simulink model "PMSM_FOC_Speed_PR"  (R2024b)
settings: Solver=FixedStepAuto  StartTime=0.0  StopTime=1  FixedStep=1e-6  RelTol=1e-3
model workspace (MAT data in the model file):
  B = 0
  Current_Filter_On = 0
  F = 10000
  J = 5.8e-05
  Ls = 0.0005125
  PR_ki = 150
  PR_wc = 150
  Pn = 5
  Rs = 0.1445
  T_deadband = 3e-06
  Ts = 5e-05
  Vdc = 60
  id_ki = 0.8
  id_kp = 0.6
  iq_ki = 0.8
  iq_kp = 0.7
  psi_f = 0.0113
  speed_ki = 1.2
  speed_kp = 0.7
undefined symbols (not defined in the file): sigbuilder_block
libraries: simulink x2, spsDCVoltageSourceLib x1, spsOnDelayLib x1, spsPermanentMagnetSynchronousMachineLib x1, slpidlib x1, spsTwoLevelConverterLib x1, spspowerguiLib x1
settings Model: Creator=A  LastModifiedBy=31904
settings OptimizationCC: ReuseModelBlockBuffer=off
settings ModelReferenceCC: EnableRefExpFcnMdlSchedulingChecks=on
settings RTWCC: GPUComputeCapability=3.5

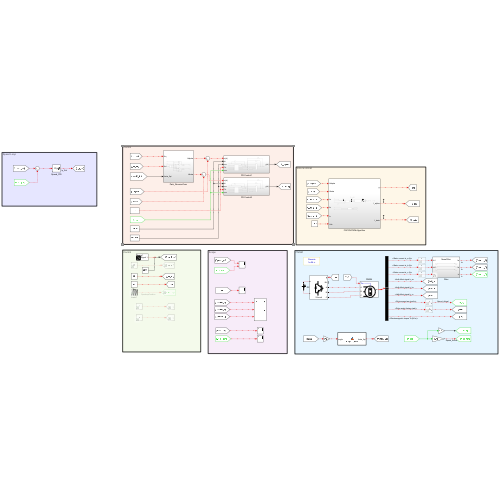
[thumbnail: Simulink's stored preview of the top-level diagram]
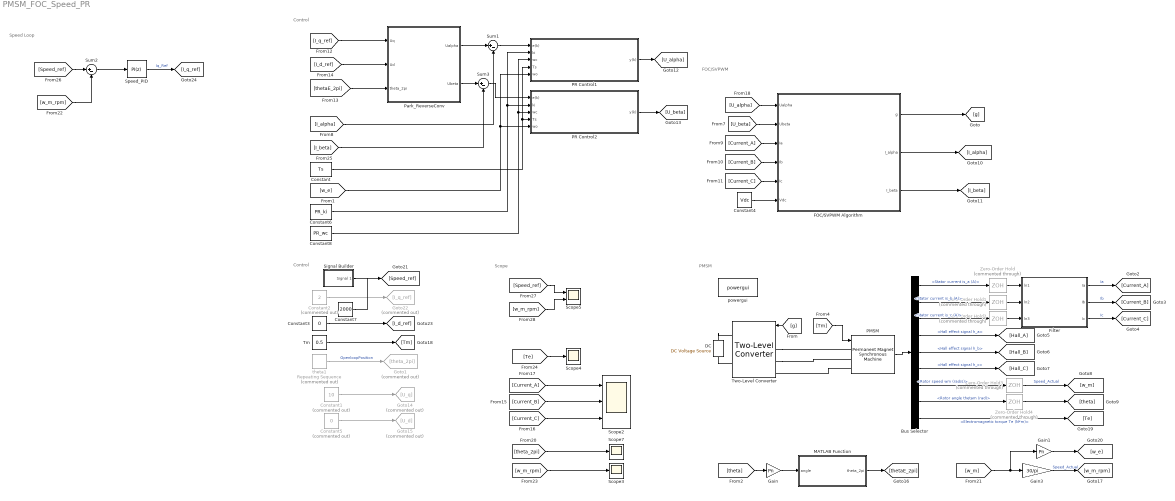
== system PMSM_FOC_Speed_PR ==
  note: Speed Loop
  note: Control
  note: Scope
  note: Control
  note: FOC/SVPWM
  note: PMSM
  Bus Selector : BusSelector  OutputSignals=Stator current is_a (A),Stator current is_b (A),Stator current is_c (A),Hall effect signal h_a,Hall effect signal h_b,Hall effect signal h_c,Rotor speed wm (rad/s),Rotor angle thetam (rad),Electromagnetic torque Te (N*m)
  Constant : Constant  Value=Ts
  Constant1 : Constant  Commented=on  Value=10
  Constant2 : Constant  Commented=on  Value=2
  Constant3 : Constant  Value=0
  Constant4 : Constant  Value=Vdc
  Constant5 : Constant  Commented=on  Value=0
  Constant6 : Constant  Value=PR_ki
  Constant7 : Constant  Value=2000
  Constant8 : Constant  Value=PR_wc
  DC : spsDCVoltageSourceLib/DC Voltage Source  Amplitude=Vdc  Measurements=None
  FOC/SVPWM Algorithm : Subsystem
  Filter : Subsystem  Variant=on
  Gain : Gain  Gain=Pn
  Gain1 : Gain  Gain=Pn
  Gain3 : Gain  Gain=30/pi
  Goto1 : Goto  Commented=on  GotoTag=theta_2pi
  Goto14 : Goto  Commented=on  GotoTag=U_q
  Goto15 : Goto  Commented=on  GotoTag=U_d
  Goto22 : Goto  Commented=on  GotoTag=I_q_ref
  MATLAB Function : MATLAB Function  TreatAsAtomicUnit=on
  PMSM : spsPermanentMagnetSynchronousMachineLib/Permanent Magnet Synchronous Machine  NbPhases=3  FluxDistribution=Sinusoidal  RotorType=Round  MechanicalLoad=Torque Tm  PresetModel=No  ShowDetailedParameters=on  MeasurementBus=off  Resistance=Rs  Inductance=8.5e-3  dqInductances=[8.5e-3,8.5e-3]  La=Ls  MachineConstant=Flux linkage established by magnets (V.s)  Flux=psi_f  VoltageCst=10.248  TorqueCst=0.08475  Flat=120  Mechanical=[J B Pn 0]  PolePairs=4  InitialConditions=[0,0, 0,0]  InitialConditions5ph=[0 0 0 0 0 0]  RefAngle=Aligned with phase A axis (original Park)  IterativeDiscreteModel=Trapezoidal non iterative  TsBlock=-1  TsPowergui=0
  PR Control1 : Subsystem
  PR Control2 : Subsystem
  Park_ReverseConv : Subsystem
  Scope2 : Scope  NumInputPorts=3
  Scope3 : Scope
  Scope4 : Scope
  Scope5 : Scope  NumInputPorts=2
  Scope7 : Scope
  Signal Builder : Subsystem  Tag=STV Subsys  LoadFcn=sigbuilder_block('load');  StartFcn=sigbuilder_block('start');  StopFcn=sigbuilder_block('stop');  ClipboardFcn=sigbuilder_block('clipboard');  mask(Sigbuilder block){tuvar=[0:10]}
      mask help: Simulink:masks:SigbuilderBlock_MD
      mask init:
      | if ~strcmp(get_param(bdroot(gcbh),'SimulationStatus'),'stopped') tuvar = sigbuilder_block('maskInit'); end
      settings: CopyFcn=sigbuilder_block('copy');  DeleteFcn=sigbuilder_block('delete');  ModelCloseFcn=sigbuilder_block('modelClose');  PreSaveFcn=sigbuilder_block('preSave');  PauseFcn=sigbuilder_block('pause');  ContinueFcn=sigbuilder_block('continue');  NameChangeFcn=sigbuilder_block('namechange');  OpenFcn=sigbuilder_block('open',[458.1 40.8 550.2 399.9 ]);  CloseFcn=sigbuilder_block('close');
      mask Display: plot(0, 0, 100, 100,[2, 2, 32, 32, 2], [68, 8, 8, 68, 68],[32, 2], [38, 38], [32, 19, 2],[53, 60, 44], [32, 17, 17, 2],[16, 16, 31, 31]);txt = getActiveGroup(gcbh);text(2, 100, txt,'verticalAlignment', 'top');
  Speed_PID : slpidlib/PID Controller  Controller=PI  Form=Parallel  TimeDomain=Discrete-time  UseExternalTs=off  SampleTime=-1  IntegratorMethod=Forward Euler  FilterMethod=Forward Euler  ControllerParametersSource=internal  P=speed_kp  I=speed_ki  UseKiTs=off  D=0  UseExternalDerivativeSource=off  N=100  UseFilter=on  TunerSelectOption=Transfer Function Based (PID Tuner App)  InitialConditionSource=internal  InitialConditionForIntegrator=0  InitialConditionForFilter=0  DifferentiatorICPrevScaledInput=0  ExternalReset=none  TrackingMode=off  Kt=1  LimitOutput=on  SatLimitsSource=internal  UpperSaturationLimit=Vdc  LowerSaturationLimit=-Vdc  LinearizeAsGain=on  AntiWindupMode=back-calculation  Kb=0.5  LimitIntegrator=off  UpperIntegratorSaturationLimit=inf  LowerIntegratorSaturationLimit=-inf  POutMin=[]  POutMax=[]  IOutMin=[]  IOutMax=[]  DOutMin=[]  DOutMax=[]  NOutMin=[]  NOutMax=[]  SumOutMin=[]  SumOutMax=[]  SaturationOutMin=[]  SaturationOutMax=[]  PParamMin=[]  PParamMax=[]  IParamMin=[]  IParamMax=[]  DParamMin=[]  DParamMax=[]  NParamMin=[]  NParamMax=[]  KbParamMin=[]  KbParamMax=[]  KtParamMin=[]  KtParamMax=[]  KbOutMin=[]  KbOutMax=[]  KtOutMin=[]  KtOutMax=[]  IntegratorOutMin=[]  IntegratorOutMax=[]  FilterOutMin=[]  FilterOutMax=[]  SumI1OutMin=[]  SumI1OutMax=[]  SumI2OutMin=[]  SumI2OutMax=[]  SumI3OutMin=[]  SumI3OutMax=[]  SumI4OutMin=[]  SumI4OutMax=[]  SumDOutMin=[]  SumDOutMax=[]  DifferentiatorOutMin=[]  DifferentiatorOutMax=[]  FilterDiffOutCoefMin=[]  FilterDiffOutCoefMax=[]  ReciprocalOutMin=[]  ReciprocalOutMax=[]  SumDenOutMin=[]  SumDenOutMax=[]  SumNumOutMin=[]  SumNumOutMax=[]  DivideOutMin=[]  DivideOutMax=[]  UdiffTsProdOutMin=[]  UdiffTsProdOutMax=[]  NTsProdOutMin=[]  NTsProdOutMax=[]  UintegralTsProdOutMin=[]  UintegralTsProdOutMax=[]  UngainTsProdOutMin=[]  UngainTsProdOutMax=[]  ClampingZeroOutDataTypeStr=Inherit: Inherit via back propagation  ClampingZeroOutMin=[]  ClampingZeroOutMax=[]  FilterDenConstantOutDataTypeStr=Inherit: Inherit via back propagation  FilterDenConstantOutMin=[]  FilterDenConstantOutMax=[]  PCopyOutDataTypeStr=Inherit: Inherit via back propagation  PCopyOutMin=[]  PCopyOutMax=[]  NCopyOutDataTypeStr=Inherit: Inherit via back propagation  NCopyOutMin=[]  NCopyOutMax=[]  IntegratorContinuousStateAttributes=''  IntegratorStateMustResolveToSignalObject=off  IntegratorRTWStateStorageClass=Auto  FilterContinuousStateAttributes=''  FilterStateMustResolveToSignalObject=off  FilterRTWStateStorageClass=Auto  ParallelPVariant=InternalParameters  IdealPVariant=Disabled  IVariant=InternalParameters  DVariant=Disabled  IntegratorVariant=Discrete  SatVariant=Enabled  AWVariant=BackCalculation  PCopyVariant=Disabled  TRVariant=Disabled  FdbkBlocksVariant=Forward  IdealPFdbkVariant=Disabled  SatFdbkVariant=Disabled  DerivativeFilterVariant=Disabled  NVariant=Disabled  NCopyVariant=Disabled_SignalSpec  FilterICVariant=Disabled  IntegratorICVariant=InternalICs  ExternalResetVariant=Disabled  TRSumVariant=Passthrough  SumFdbkVariant=Disabled  SumVariant=Sum_PI  TsampFilterVariant=InternalTs  TsampNgainVariant=Passthrough  TsampIntegralVariant=Disabled_SignalSpec  ExternalSaturationOutDataTypeStr=Inherit: Same as second input  DerivativeSourceVariant=Disabled  PreIntVariant=InternalPreInt
  Sum1 : Sum  Inputs=|+-
  Sum2 : Sum  Inputs=|+-
  Sum3 : Sum  Inputs=|+-
  Tm : Constant  Value=0.5
  Two-Level Converter : spsTwoLevelConverterLib/Two-Level Converter  ModelType=Switching devices  Ron=1e-3  Rs=1e6  Cs=inf  Vforward=[0,0]  Ron_Diode=1e-3  Rs_Diode=1e6  Cs_Diode=inf  Vf_Diode=1e-3  Rs_CurrentSource=inf  Ron_ACsource=1e-3
  Zero-Order Hold{,1..4} (5 alike) : ZeroOrderHold  Commented=through  SampleTime=1/F
  powergui : spspowerguiLib/powergui  Priority=1  SimulationMode=Discrete  SampleTime=1e-6  frequency=60  Iterations=50  frequencyindice=0  Pbase=100e6  ErrMax=1e-4  UnitsV=kV  UnitsW=MW  buscounter=0  FunctionMessages=off  echomessages=off  EnableUseOfTLC=off  CurrentSourceSwitches=off  DisableSnubberDevices=off  DisableRonSwitches=off  DisableVfSwitches=off  DisplayEquations=off  AutomaticDiscreteSolvers=off  SolverType=Tustin/Backward Euler (TBE)  Interpol=off  ExternalGateDelay=off  methode=off  Ts=100  x0status=blocks  SPID=on  SwTol=0  HookPort=off  NonlinearTolerance=1e-4  nMaxIteration=100  ContinueOnMaxIteration=off  RestoreLinks=warning  ResistiveCurrentMeasurement=off  Frange=[0:2:500]  Ylog=off  Xlog=on  ShowGrid=off  save=off  variable=ZData  structure=0  ZoomFFT=off  StartTime=0.0  cycles=1  DisplayStyle=1  fundamental=60  FreqAxis=off  MaxFrequency=1000  frequencyindicesteady=1  RmsSteady=1  display=off
  theta1 : simulink/Sources/Repeating Sequence  Commented=on  rep_seq_t=[0 0.1]  rep_seq_y=[0 2*pi]
  wires:
  Constant4/1 -> FOC/SVPWM Algorithm/6(Vdc)
  FOC/SVPWM Algorithm/3(I_beta) -> [I_beta]
  [U_beta] -> FOC/SVPWM Algorithm/2(Ubeta)
  [U_alpha] -> FOC/SVPWM Algorithm/1(Ualpha)
  [Current_A] -> FOC/SVPWM Algorithm/3(Ia)
  [Current_C] -> FOC/SVPWM Algorithm/5(Ic)
  FOC/SVPWM Algorithm/2(I_alpha) -> [I_alpha]
  [Current_B] -> FOC/SVPWM Algorithm/4(Ib)
  Zero-Order Hold4/1 -> [theta]
  Bus Selector/1 -> Zero-Order Hold/1  "<Stator current is_a (A)>"
  Zero-Order Hold/1 -> Filter/1(ln1)
  Zero-Order Hold1/1 -> Filter/2(ln2)
  Bus Selector/4 -> [Hall_A]  "<Hall effect signal h_a>"
  [theta] -> Gain/1
  Bus Selector/2 -> Zero-Order Hold1/1  "<Stator current is_b (A)>"
  [g] -> Two-Level Converter/1
  Bus Selector/3 -> Zero-Order Hold2/1  "<Stator current is_c (A)>"
  [Tm] -> PMSM/1
  Zero-Order Hold3/1 -> [w_m]  "Speed_Actual"
  Bus Selector/8 -> Zero-Order Hold4/1  "<Rotor angle thetam (rad)>"
  MATLAB Function/1(theta_2pi) -> [thetaE_2pi]
  Bus Selector/7 -> Zero-Order Hold3/1  "<Rotor speed wm (rad/s)>"
  PMSM/1 -> Bus Selector/1
  Bus Selector/5 -> [Hall_B]  "<Hall effect signal h_b>"
  Zero-Order Hold2/1 -> Filter/3(ln3)
  Bus Selector/6 -> [Hall_C]  "<Hall effect signal h_c>"
  Constant3/1 -> [I_d_ref]
  Constant2/1 -> Goto22/1
  [I_q_ref] -> Park_ReverseConv/1(Uq)
  [Current_C] -> Scope2/3
  [Current_B] -> Scope2/2
  [Current_A] -> Scope2/1
  [theta_2pi] -> Scope7/1
  Filter/1(Ia) -> [Current_A]  "Ia"
  Filter/2(Ib) -> [Current_B]  "Ib"
  Filter/3(Ic) -> [Current_C]  "Ic"
  FOC/SVPWM Algorithm/1(g) -> [g]
  theta1/1 -> Goto1/1  "OpenloopPosition"
  [I_d_ref] -> Park_ReverseConv/2(Ud)
  Constant5/1 -> Goto15/1
  Constant1/1 -> Goto14/1
  [w_m] -> Gain1/1, Gain3/1
  Gain3/1 -> [w_m_rpm]  "Speed_Actual"
  [w_m_rpm] -> Scope3/1
  Gain/1 -> MATLAB Function/1(angle)
  Tm/1 -> [Tm]
  Bus Selector/9 -> [Te]  "<Electromagnetic torque Te (N*m)>"
  [Te] -> Scope4/1
  PR Control2/1(y(k)) -> [U_beta]
  PR Control1/1(y(k)) -> [U_alpha]
  Constant7/1 -> [Speed_ref]
  Sum2/1 -> Speed_PID/1
  [w_m_rpm] -> Sum2/2
  [Speed_ref] -> Sum2/1
  Speed_PID/1 -> [I_q_ref]  "Iq_Ref"
  [Speed_ref] -> Scope5/1
  [w_m_rpm] -> Scope5/2
  Signal Builder/1(Signal 1) -> ?
  [thetaE_2pi] -> Park_ReverseConv/3(theta_2pi)
  Park_ReverseConv/1(Ualpha) -> Sum1/1
  Park_ReverseConv/2(Ubeta) -> Sum3/1
  Sum1/1 -> PR Control1/1(e(k))
  [I_alpha] -> Sum1/2
  [I_beta] -> Sum3/2
  Sum3/1 -> PR Control2/1(e(k))
  Constant/1 -> PR Control1/4(Ts), PR Control2/4(Ts)
  Constant6/1 -> PR Control1/2(ki), PR Control2/2(ki)
  Constant8/1 -> PR Control1/3(wc), PR Control2/3(wc)
  Gain1/1 -> [w_e]
  [w_e] -> PR Control1/5(wo), PR Control2/5(wo)
  connections:
  DC/LConn1 -- Two-Level Converter/RConn2
  DC/RConn1 -- Two-Level Converter/RConn1
  PMSM/LConn3 -- Two-Level Converter/LConn3
  Two-Level Converter/LConn1 -- PMSM/LConn1
  Two-Level Converter/LConn2 -- PMSM/LConn2

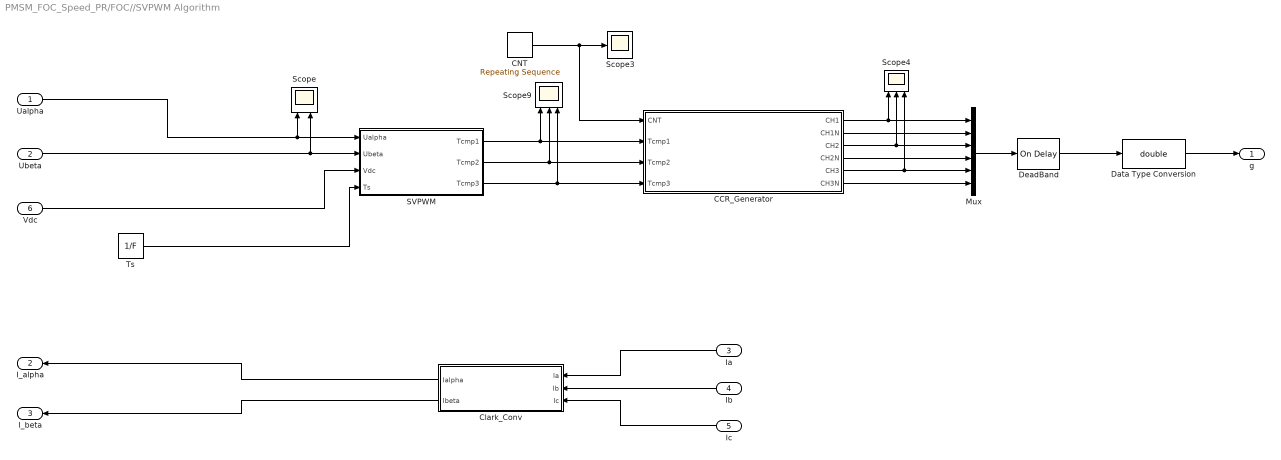
== system PMSM_FOC_Speed_PR/FOC//SVPWM Algorithm ==
  Ualpha : Inport
  Ubeta : Inport  Port=2
  Ia : Inport  Port=3
  Ib : Inport  Port=4
  Ic : Inport  Port=5
  Vdc : Inport  Port=6
  CCR_Generator : MATLAB Function  TreatAsAtomicUnit=on
  CNT : simulink/Sources/Repeating Sequence  rep_seq_t=[0 1/(2*F) 1/F]  rep_seq_y=[0 1/(2*F) 0]
  Clark_Conv : Subsystem
  Data Type Conversion : DataTypeConversion  OutDataTypeStr=double  SaturateOnIntegerOverflow=off  RndMeth=Floor
  DeadBand : spsOnDelayLib/On Delay  DelayType=On delay  delay=T_deadband  ic=0  Ts=0
  Mux : Mux  Inputs=6
  SVPWM : Subsystem
  Scope : Scope  NumInputPorts=2
  Scope3 : Scope
  Scope4 : Scope  NumInputPorts=3
  Scope9 : Scope  NumInputPorts=3
  Ts : Constant  Value=1/F
  g : Outport
  I_alpha : Outport  Port=2
  I_beta : Outport  Port=3
  wires:
  SVPWM/3(Tcmp3) -> CCR_Generator/4(Tcmp3), Scope9/3
  Clark_Conv/1(Ialpha) -> I_alpha/1
  CCR_Generator/3(CH2) -> Mux/3, Scope4/2
  SVPWM/2(Tcmp2) -> CCR_Generator/3(Tcmp2), Scope9/2
  CCR_Generator/2(CH1N) -> Mux/2
  CCR_Generator/5(CH3) -> Mux/5, Scope4/3
  SVPWM/1(Tcmp1) -> CCR_Generator/2(Tcmp1), Scope9/1
  Clark_Conv/2(Ibeta) -> I_beta/1
  CCR_Generator/4(CH2N) -> Mux/4
  Ualpha/1 -> SVPWM/1(Ualpha), Scope/1
  CCR_Generator/6(CH3N) -> Mux/6
  Mux/1 -> DeadBand/1
  Ubeta/1 -> Scope/2, SVPWM/2(Ubeta)
  CNT/1 -> Scope3/1, CCR_Generator/1(CNT)
  CCR_Generator/1(CH1) -> Mux/1, Scope4/1
  Data Type Conversion/1 -> g/1
  Vdc/1 -> SVPWM/3(Vdc)
  Ic/1 -> Clark_Conv/3(Ic)
  Ib/1 -> Clark_Conv/2(Ib)
  Ia/1 -> Clark_Conv/1(Ia)
  Ts/1 -> SVPWM/4(Ts)
  DeadBand/1 -> Data Type Conversion/1

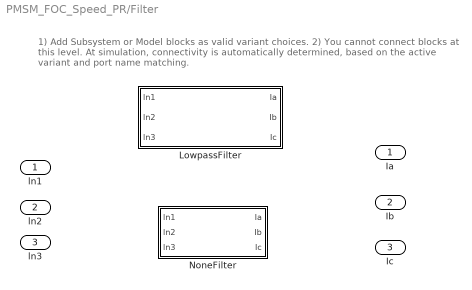
== system PMSM_FOC_Speed_PR/Filter ==
  note: 1) Add Subsystem or Model blocks as valid variant choices.
      | 2) You cannot connect blocks at this level. At simulation, connectivity is automatically
      | determined, based on the active variant and port name matching.
  ln1 : Inport
  ln2 : Inport  Port=2
  ln3 : Inport  Port=3
  LowpassFilter : Subsystem  VariantControl=Current_Filter_On==1
  NoneFilter : Subsystem  VariantControl=Current_Filter_On==0
  Ia : Outport
  Ib : Outport  Port=2
  Ic : Outport  Port=3

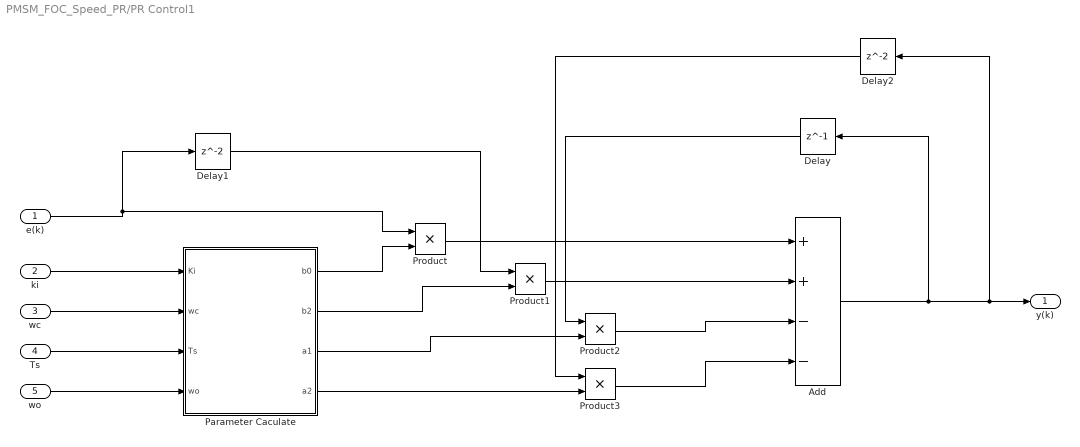
== system PMSM_FOC_Speed_PR/PR Control1 ==
  e(k) : Inport
  ki : Inport  Port=2
  wc : Inport  Port=3
  Ts : Inport  Port=4
  wo : Inport  Port=5
  Add : Sum  Inputs=++--
  Delay : Delay  DelayLength=1  InputProcessing=Columns as channels (frame based)
  Delay1 : Delay  InputProcessing=Columns as channels (frame based)
  Delay2 : Delay  InputProcessing=Columns as channels (frame based)
  Parameter Caculate : MATLAB Function  TreatAsAtomicUnit=on
  Product{,1..3} (4 alike) : Product
  y(k) : Outport
  wires:
  Ts/1 -> Parameter Caculate/3(Ts)
  wc/1 -> Parameter Caculate/2(wc)
  wo/1 -> Parameter Caculate/4(wo)
  Product2/1 -> Add/3
  ki/1 -> Parameter Caculate/1(Ki)
  Parameter Caculate/4(a2) -> Product3/2
  Delay2/1 -> Product3/1
  Parameter Caculate/1(b0) -> Product/2
  Delay/1 -> Product2/1
  Parameter Caculate/2(b2) -> Product1/2
  Add/1 -> Delay2/1, y(k)/1, Delay/1
  Product3/1 -> Add/4
  Product/1 -> Add/1
  Product1/1 -> Add/2
  e(k)/1 -> Product/1, Delay1/1
  Delay1/1 -> Product1/1
  Parameter Caculate/3(a1) -> Product2/2

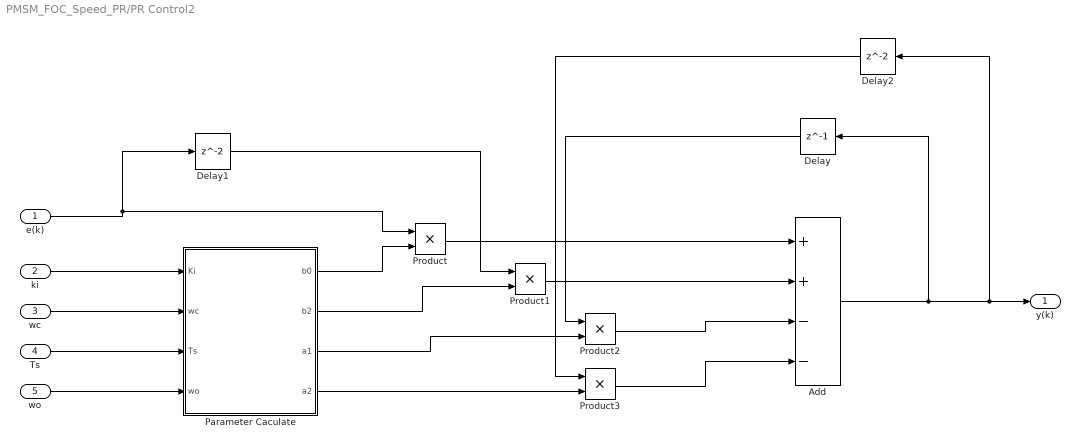
== system PMSM_FOC_Speed_PR/PR Control2 ==
  e(k) : Inport
  ki : Inport  Port=2
  wc : Inport  Port=3
  Ts : Inport  Port=4
  wo : Inport  Port=5
  Add : Sum  Inputs=++--
  Delay : Delay  DelayLength=1  InputProcessing=Columns as channels (frame based)
  Delay1 : Delay  InputProcessing=Columns as channels (frame based)
  Delay2 : Delay  InputProcessing=Columns as channels (frame based)
  Parameter Caculate : MATLAB Function  TreatAsAtomicUnit=on
  Product{,1..3} (4 alike) : Product
  y(k) : Outport
  wires:
  Parameter Caculate/3(a1) -> Product2/2
  Delay1/1 -> Product1/1
  e(k)/1 -> Delay1/1, Product/1
  Product1/1 -> Add/2
  Product/1 -> Add/1
  Product3/1 -> Add/4
  Add/1 -> Delay/1, y(k)/1, Delay2/1
  Parameter Caculate/2(b2) -> Product1/2
  Delay/1 -> Product2/1
  Parameter Caculate/1(b0) -> Product/2
  Delay2/1 -> Product3/1
  Parameter Caculate/4(a2) -> Product3/2
  ki/1 -> Parameter Caculate/1(Ki)
  Product2/1 -> Add/3
  wo/1 -> Parameter Caculate/4(wo)
  wc/1 -> Parameter Caculate/2(wc)
  Ts/1 -> Parameter Caculate/3(Ts)

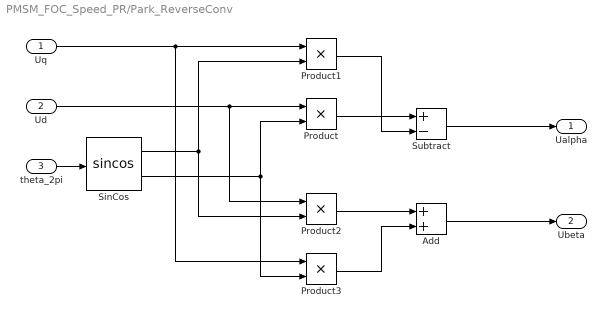
== system PMSM_FOC_Speed_PR/Park_ReverseConv ==
  Uq : Inport
  Ud : Inport  Port=2
  theta_2pi : Inport  Port=3
  Add : Sum
  Product{,1..3} (4 alike) : Product
  SinCos : Trigonometry  Operator=sincos
  Subtract : Sum  Inputs=+-
  Ualpha : Outport
  Ubeta : Outport  Port=2
  wires:
  Uq/1 -> Product3/1, Product1/1
  Ud/1 -> Product2/1, Product/1
  SinCos/2 -> Product3/2, Product/2
  Product/1 -> Subtract/1
  SinCos/1 -> Product2/2, Product1/2
  Product1/1 -> Subtract/2
  Subtract/1 -> Ualpha/1
  Product2/1 -> Add/1
  Product3/1 -> Add/2
  Add/1 -> Ubeta/1
  theta_2pi/1 -> SinCos/1

== system PMSM_FOC_Speed_PR/Signal Builder ==
  Demux : Demux  Tag=STV Demux  Outputs=1
      settings: DisplayOption=none
  FromWs : FromWorkspace  Tag=STV FromWs  VariableName=tuvar
      SigBuilderData=|
      | common.afterFinalStr = 'Extrapolate'
      | common.sampleTime = 0
      | dataSet.timeRange = [0 1]
      | dataSet.name = 'Group 1'
      | sbobj.Groups.Name = 'Group 1'
      | sbobj.Groups.Signals.Name = 'Signal 1'
      | sbobj.Groups.Signals.XData = [0 0 0.2 0.2 0.3 0.3 0.5 0.5 0.6 0.6 0.8 0.8 0.9 0.9 1]
      | sbobj.Groups.Signals.YData = [0 1000 1000 3000 3000 5000 5000 4000 4000 2000 2000 1000 1000 0 0]
      | sbobj.Groups.TimeRange = [0 1]
  Signal 1 : Outport  Tag=STV Outport
  wires:
  Demux/1 -> Signal 1/1
  FromWs/1 -> Demux/1

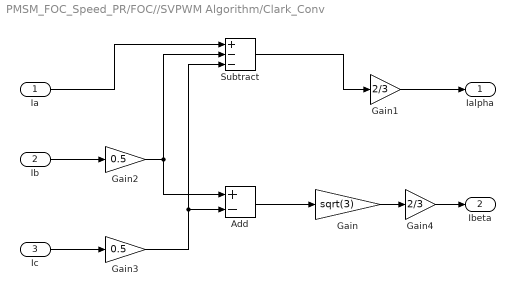
== system PMSM_FOC_Speed_PR/FOC//SVPWM Algorithm/Clark_Conv ==
  Ia : Inport
  Ib : Inport  Port=2
  Ic : Inport  Port=3
  Add : Sum  Inputs=+-  OutDataTypeStr=double
  Gain : Gain  Gain=sqrt(3)  ParamDataTypeStr=double
  Gain1 : Gain  Gain=2/3
  Gain2 : Gain  Gain=0.5
  Gain3 : Gain  Gain=0.5
  Gain4 : Gain  Gain=2/3
  Subtract : Sum  Inputs=+--  OutDataTypeStr=double
  Ialpha : Outport
  Ibeta : Outport  Port=2
  wires:
  Ia/1 -> Subtract/1
  Ib/1 -> Gain2/1
  Add/1 -> Gain/1
  Gain/1 -> Gain4/1
  Ic/1 -> Gain3/1
  Gain2/1 -> Subtract/2, Add/1
  Gain3/1 -> Subtract/3, Add/2
  Subtract/1 -> Gain1/1
  Gain1/1 -> Ialpha/1
  Gain4/1 -> Ibeta/1

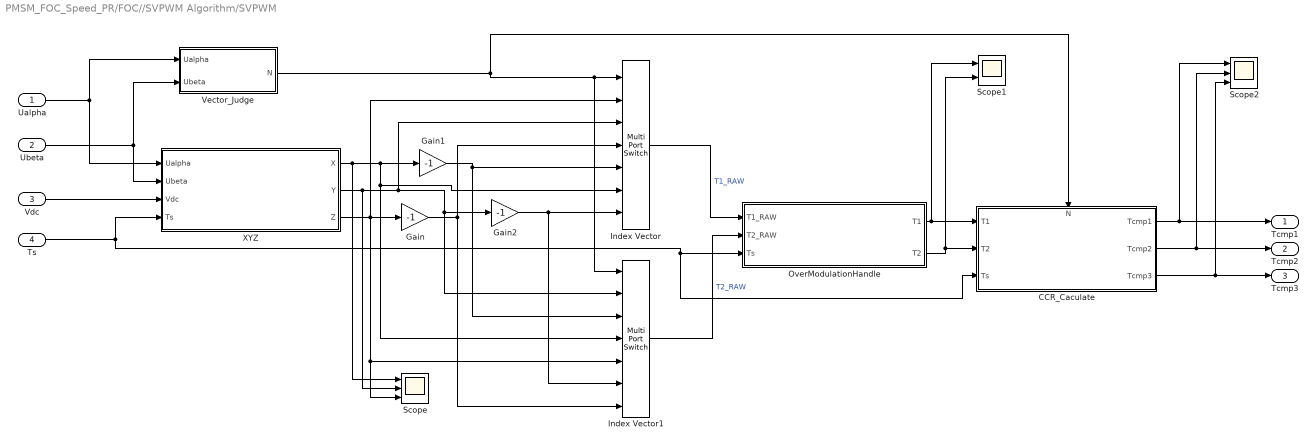
== system PMSM_FOC_Speed_PR/FOC//SVPWM Algorithm/SVPWM ==
  Ualpha : Inport
  Ubeta : Inport  Port=2
  Vdc : Inport  Port=3
  Ts : Inport  Port=4
  CCR_Caculate : Subsystem
      settings: PortSchema="{\"entries\":[{\"content\":{\"sides\":[{\"content\":{\"connectorIds\":[\"In1\",\"In2\",\"In3\"]},\"type\":\"ConnectorPlacement.EquallySpacedRectSide\",\"uuid\":\"41d89106-695f-4d7e-9c99-c52170b99868\"},{\"content\":{\"connectorIds\":[\"Out1\",\"Out2\",\"Out3\"],\"side\":\"RIGHT\"},\"type\":\"ConnectorPlacement.EquallySpacedRectSide\",\"uuid\":\"0fa1e6b9-7088-4c16-9dd3-c016449aae3e\"},{\"content\":{\"connectorIds\":[\"In4\"],\"side\":\"TOP\"},\"type\":\"ConnectorPlacement.EquallySpacedRectSide\",\"uuid\":\"6b702c00-29ab-49c7-a344-eb6fce3368af\"}]},\"type\":\"ConnectorPlacement.EquallySpacedConnector\",\"uuid\":\"c2f99839-550c-47c5-98fa-a115626cfb71\"}],\"packageUris\":[\"http://schema.mathworks.com/mf0/Connector/R2020b\"],\"version\":\"1.0\"}"
  Gain : Gain  Gain=-1
  Gain1 : Gain  Gain=-1
  Gain2 : Gain  Gain=-1
  Index Vector : MultiPortSwitch  Inputs=6  DiagnosticForDefault=None  SaturateOnIntegerOverflow=off  InputSameDT=off
  Index Vector1 : MultiPortSwitch  Inputs=6  DiagnosticForDefault=None  SaturateOnIntegerOverflow=off  InputSameDT=off
  OverModulationHandle : MATLAB Function  TreatAsAtomicUnit=on
  Scope : Scope  NumInputPorts=3
  Scope1 : Scope  NumInputPorts=2
  Scope2 : Scope  NumInputPorts=3
  Vector_Judge : Subsystem
  XYZ : Subsystem
  Tcmp1 : Outport
  Tcmp2 : Outport  Port=2
  Tcmp3 : Outport  Port=3
  wires:
  Ualpha/1 -> Vector_Judge/1(Ualpha), XYZ/1(Ualpha)
  Ubeta/1 -> Vector_Judge/2(Ubeta), XYZ/2(Ubeta)
  Vdc/1 -> XYZ/3(Vdc)
  Ts/1 -> CCR_Caculate/3(Ts), OverModulationHandle/3(Ts), XYZ/4(Ts)
  Vector_Judge/1(N) -> Index Vector1/1, Index Vector/1, CCR_Caculate/4(N)
  Index Vector1/1 -> OverModulationHandle/2(T2_RAW)  "T2_RAW"
  XYZ/3(Z) -> Scope/3, Index Vector1/5, Index Vector/2, Gain/1
  XYZ/2(Y) -> Scope/2, Index Vector1/2, Gain2/1, Index Vector/3
  Gain/1 -> Index Vector1/7, Index Vector/4
  XYZ/1(X) -> Scope/1, Index Vector1/4, Index Vector/6, Gain1/1
  Gain1/1 -> Index Vector1/3, Index Vector/5
  Gain2/1 -> Index Vector1/6, Index Vector/7
  Index Vector/1 -> OverModulationHandle/1(T1_RAW)  "T1_RAW"
  OverModulationHandle/1(T1) -> CCR_Caculate/1(T1), Scope1/1
  OverModulationHandle/2(T2) -> Scope1/2, CCR_Caculate/2(T2)
  CCR_Caculate/1(Tcmp1) -> Tcmp1/1, Scope2/1
  CCR_Caculate/2(Tcmp2) -> Tcmp2/1, Scope2/2
  CCR_Caculate/3(Tcmp3) -> Tcmp3/1, Scope2/3

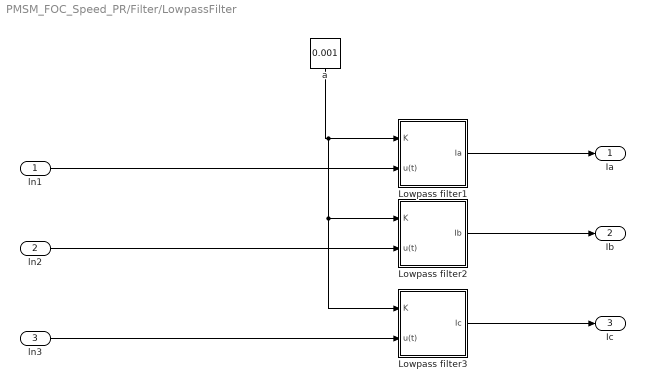
== system PMSM_FOC_Speed_PR/Filter/LowpassFilter ==
  ln1 : Inport
  ln2 : Inport  Port=2
  ln3 : Inport  Port=3
  Lowpass filter1 : Subsystem
  Lowpass filter2 : Subsystem
  Lowpass filter3 : Subsystem
  a : Constant  Value=0.001
  Ia : Outport
  Ib : Outport  Port=2
  Ic : Outport  Port=3
  wires:
  ln2/1 -> Lowpass filter2/2(u(t))
  a/1 -> Lowpass filter3/1(K), Lowpass filter2/1(K), Lowpass filter1/1(K)
  ln1/1 -> Lowpass filter1/2(u(t))
  Lowpass filter1/1(Ia) -> Ia/1
  Lowpass filter2/1(Ib) -> Ib/1
  Lowpass filter3/1(Ic) -> Ic/1
  ln3/1 -> Lowpass filter3/2(u(t))

== system PMSM_FOC_Speed_PR/Filter/NoneFilter ==
  ln1 : Inport
  ln2 : Inport  Port=2
  ln3 : Inport  Port=3
  Ia : Outport
  Ib : Outport  Port=2
  Ic : Outport  Port=3
  wires:
  ln1/1 -> Ia/1
  ln2/1 -> Ib/1
  ln3/1 -> Ic/1

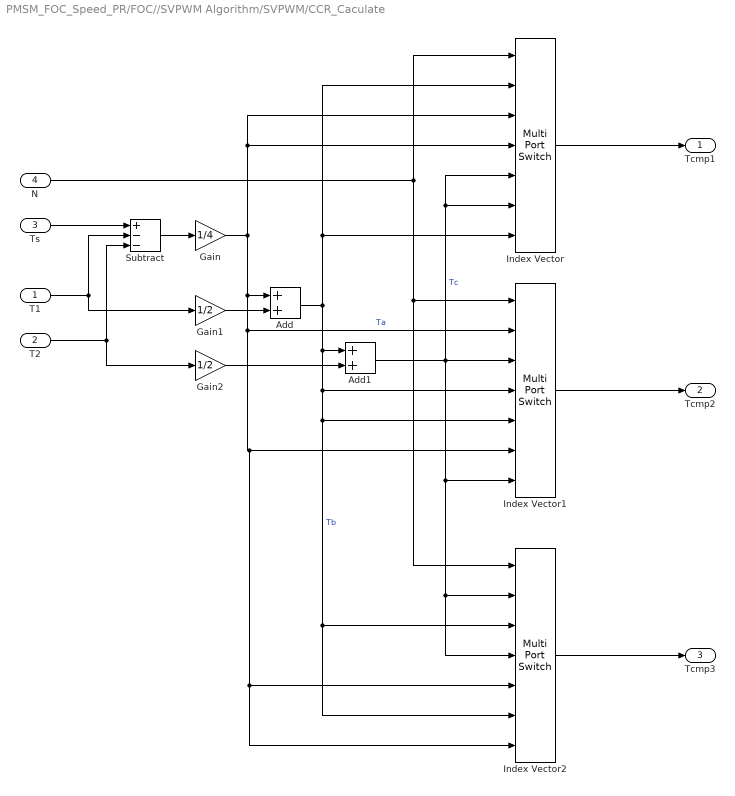
== system PMSM_FOC_Speed_PR/FOC//SVPWM Algorithm/SVPWM/CCR_Caculate ==
  T1 : Inport
  T2 : Inport  Port=2
  Ts : Inport  Port=3
  N : Inport  Port=4
  Add : Sum
  Add1 : Sum
  Gain : Gain  Gain=1/4
  Gain1 : Gain  Gain=1/2
  Gain2 : Gain  Gain=1/2
  Index Vector : MultiPortSwitch  Inputs=6  DiagnosticForDefault=None  SaturateOnIntegerOverflow=off  InputSameDT=off
  Index Vector1 : MultiPortSwitch  Inputs=6  DiagnosticForDefault=None  SaturateOnIntegerOverflow=off  InputSameDT=off
  Index Vector2 : MultiPortSwitch  Inputs=6  DiagnosticForDefault=None  SaturateOnIntegerOverflow=off  InputSameDT=off
  Subtract : Sum  Inputs=+--
  Tcmp1 : Outport
  Tcmp2 : Outport  Port=2
  Tcmp3 : Outport  Port=3
  wires:
  Ts/1 -> Subtract/1
  T1/1 -> Gain1/1, Subtract/2
  T2/1 -> Gain2/1, Subtract/3
  Subtract/1 -> Gain/1
  Gain/1 -> Index Vector2/7, Index Vector2/5, Index Vector1/6, Index Vector1/2, Add/1, Index Vector/4, Index Vector/3  "Ta"
  Gain1/1 -> Add/2
  Add/1 -> Index Vector1/5, Index Vector2/6, Index Vector2/3, Index Vector1/4, Add1/1, Index Vector/7, Index Vector/2  "Tb"
  Gain2/1 -> Add1/2
  Add1/1 -> Index Vector2/4, Index Vector2/2, Index Vector1/7, Index Vector1/3, Index Vector/6, Index Vector/5  "Tc"
  N/1 -> Index Vector2/1, Index Vector1/1, Index Vector/1
  Index Vector/1 -> Tcmp1/1
  Index Vector1/1 -> Tcmp2/1
  Index Vector2/1 -> Tcmp3/1

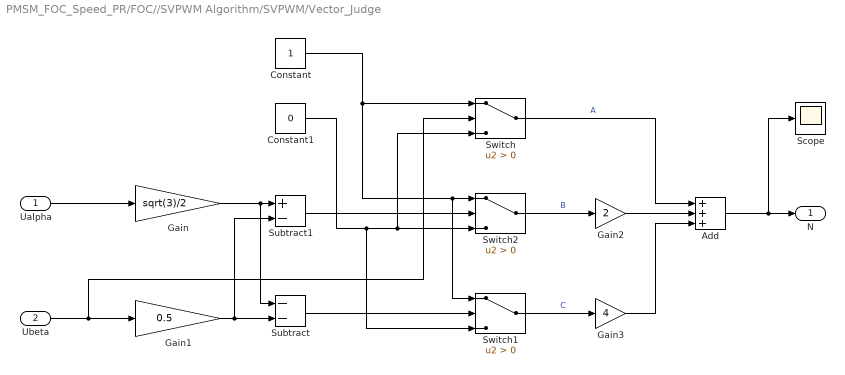
== system PMSM_FOC_Speed_PR/FOC//SVPWM Algorithm/SVPWM/Vector_Judge ==
  Ualpha : Inport
  Ubeta : Inport  Port=2
  Add : Sum  Inputs=+++
  Constant : Constant
  Constant1 : Constant  Value=0
  Gain : Gain  Gain=sqrt(3)/2
  Gain1 : Gain  Gain=0.5
  Gain2 : Gain  Gain=2
  Gain3 : Gain  Gain=4
  Scope : Scope
  Subtract : Sum  Inputs=--
  Subtract1 : Sum  Inputs=+-
  Switch : Switch  Criteria=u2 > Threshold  SaturateOnIntegerOverflow=off  InputSameDT=off
  Switch1 : Switch  Criteria=u2 > Threshold  SaturateOnIntegerOverflow=off  InputSameDT=off
  Switch2 : Switch  Criteria=u2 > Threshold  SaturateOnIntegerOverflow=off  InputSameDT=off
  N : Outport
  wires:
  Ualpha/1 -> Gain/1
  Ubeta/1 -> Gain1/1, Switch/2
  Switch/1 -> Add/1  "A"
  Switch1/1 -> Gain3/1  "C"
  Constant1/1 -> Switch2/3, Switch/3, Switch1/3
  Constant/1 -> Switch2/1, Switch1/1, Switch/1
  Switch2/1 -> Gain2/1  "B"
  Gain3/1 -> Add/3
  Add/1 -> Scope/1, N/1
  Gain2/1 -> Add/2
  Gain/1 -> Subtract/1, Subtract1/1
  Gain1/1 -> Subtract/2, Subtract1/2
  Subtract1/1 -> Switch2/2
  Subtract/1 -> Switch1/2

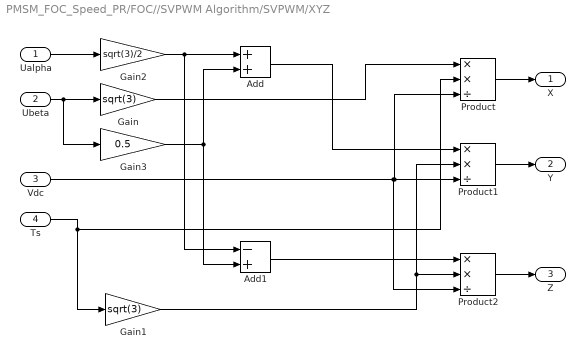
== system PMSM_FOC_Speed_PR/FOC//SVPWM Algorithm/SVPWM/XYZ ==
  Ualpha : Inport
  Ubeta : Inport  Port=2
  Vdc : Inport  Port=3
  Ts : Inport  Port=4
  Add : Sum
  Add1 : Sum  Inputs=-+
  Gain : Gain  Gain=sqrt(3)
  Gain1 : Gain  Gain=sqrt(3)
  Gain2 : Gain  Gain=sqrt(3)/2
  Gain3 : Gain  Gain=0.5
  Product : Product  Inputs=**/
  Product1 : Product  Inputs=**/
  Product2 : Product  Inputs=**/
  X : Outport
  Y : Outport  Port=2
  Z : Outport  Port=3
  wires:
  Ualpha/1 -> Gain2/1
  Gain/1 -> Product/1
  Ubeta/1 -> Gain3/1, Gain/1
  Ts/1 -> Product/2, Gain1/1
  Vdc/1 -> Product1/3, Product/3, Product2/3
  Product/1 -> X/1
  Gain2/1 -> Add1/1, Add/1
  Gain3/1 -> Add/2, Add1/2
  Add/1 -> Product1/1
  Gain1/1 -> Product2/2, Product1/2
  Product1/1 -> Y/1
  Add1/1 -> Product2/1
  Product2/1 -> Z/1

== system PMSM_FOC_Speed_PR/Filter/LowpassFilter/Lowpass filter1 ==
  K : Inport
  u(t) : Inport  Port=2
  Add : Sum
  Delay : Delay  DelayLength=1
  Product : Product
  Subtract : Sum  Inputs=+-
  Ia : Outport
  wires:
  Add/1 -> Ia/1, Delay/1
  Product/1 -> Add/1
  Subtract/1 -> Product/2
  Delay/1 -> Subtract/2, Add/2
  K/1 -> Product/1
  u(t)/1 -> Subtract/1

== system PMSM_FOC_Speed_PR/Filter/LowpassFilter/Lowpass filter2 ==
  K : Inport
  u(t) : Inport  Port=2
  Add : Sum
  Delay : Delay  DelayLength=1
  Product : Product
  Subtract : Sum  Inputs=+-
  Ib : Outport
  wires:
  u(t)/1 -> Subtract/1
  K/1 -> Product/1
  Delay/1 -> Add/2, Subtract/2
  Subtract/1 -> Product/2
  Product/1 -> Add/1
  Add/1 -> Delay/1, Ib/1

== system PMSM_FOC_Speed_PR/Filter/LowpassFilter/Lowpass filter3 ==
  K : Inport
  u(t) : Inport  Port=2
  Add : Sum
  Delay : Delay  DelayLength=1
  Product : Product
  Subtract : Sum  Inputs=+-
  Ic : Outport
  wires:
  Add/1 -> Ic/1, Delay/1
  Product/1 -> Add/1
  Subtract/1 -> Product/2
  Delay/1 -> Subtract/2, Add/2
  K/1 -> Product/1
  u(t)/1 -> Subtract/1

== matlab function PMSM_FOC_Speed_PR/MATLAB Function ==
  data: angle input; theta_2pi output
function theta_2pi = Angle_Conv(angle)

theta_2pi=mod(angle,2*pi);

== matlab function PMSM_FOC_Speed_PR/FOC//SVPWM Algorithm/CCR_Generator ==
  data: CNT input; Tcmp1 input; Tcmp2 input; Tcmp3 input; CH1 output; CH1N output; CH2 output; CH2N output; CH3 output; CH3N output
function[CH1,CH1N,CH2,CH2N,CH3,CH3N] = CCR_Generator(CNT,Tcmp1, Tcmp2, Tcmp3)

if (CNT<Tcmp1)
    CH1=0;
    CH1N=1;
else
    CH1=1;
    CH1N=0;
end
if (CNT<Tcmp2)
    CH2=0;
    CH2N=1;
else
    CH2=1;
    CH2N=0;
end
if (CNT<Tcmp3)
    CH3=0;
    CH3N=1;
else
    CH3=1;
    CH3N=0;
end
end

== matlab function PMSM_FOC_Speed_PR/FOC//SVPWM Algorithm/SVPWM/OverModulationHandle ==
  data: T1_RAW input; T2_RAW input; T1 output; T2 output; Ts input
function [T1,T2] = OverModulationHandle(T1_RAW, T2_RAW, Ts)
if((T1_RAW+T2_RAW)>Ts)
    T1=T1_RAW/(T1_RAW+T2_RAW)*Ts;
    T2=T2_RAW/(T1_RAW+T2_RAW)*Ts;
else
    T1=T1_RAW;
    T2=T2_RAW;
end
end

== matlab function PMSM_FOC_Speed_PR/PR Control1/Parameter Caculate ==
  data: Ki input; b0 output; wc input; Ts input; wo input; b2 output; a1 output; a2 output
function [b0,b2,a1,a2] = fcn(Ki,wc,Ts,wo)
b0 = 4*Ki*wc*Ts/(4+4*wc*Ts+wo^2*Ts^2);
b2 = -4*Ki*wc*Ts/(4+4*wc*Ts+wo^2*Ts^2);
a1=(2*wo^2*Ts^2-8)/(4+4*wc*Ts+wo^2*Ts^2);
a2=(4-4*wc*Ts+wo^2*Ts^2)/(4+4*wc*Ts+wo^2*Ts^2);

== matlab function PMSM_FOC_Speed_PR/PR Control2/Parameter Caculate ==
  data: Ki input; b0 output; wc input; Ts input; wo input; b2 output; a1 output; a2 output
function [b0,b2,a1,a2] = fcn(Ki,wc,Ts,wo)
b0 = 4*Ki*wc*Ts/(4+4*wc*Ts+wo^2*Ts^2);
b2 = -4*Ki*wc*Ts/(4+4*wc*Ts+wo^2*Ts^2);
a1=(2*wo^2*Ts^2-8)/(4+4*wc*Ts+wo^2*Ts^2);
a2=(4-4*wc*Ts+wo^2*Ts^2)/(4+4*wc*Ts+wo^2*Ts^2);
